simulink model "Dryden"  (R2019b)
settings: Solver=FixedStepAuto  StartTime=0.0  StopTime=1  FixedStep=1  RelTol=1e-3
undefined symbols (not defined in the file): WIND
settings Model: Creator=ibori  LastModifiedBy=Алексей
settings RTWCC: GenCodeOnly=on  PackageGeneratedCodeAndArtifacts=on

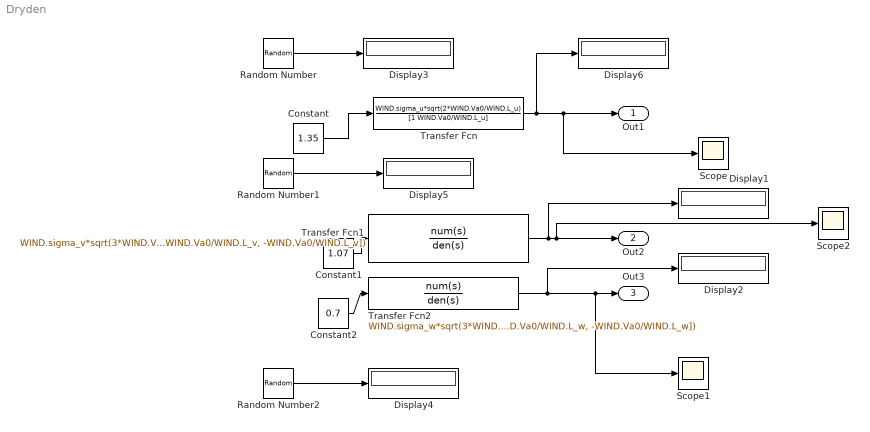
== system Dryden ==
  Constant : Constant  Value=1.35
  Constant1 : Constant  Value=1.07
  Constant2 : Constant  Value=0.7
  Display{1..6} (6 alike) : Display
  Random Number : RandomNumber  SampleTime=1
  Random Number1 : RandomNumber  SampleTime=1
  Random Number2 : RandomNumber  SampleTime=1
  Scope : Scope
  Scope1 : Scope
  Scope2 : Scope
  Transfer Fcn : TransferFcn  Numerator=WIND.sigma_u*sqrt(2*WIND.Va0/WIND.L_u)  Denominator=[1 WIND.Va0/WIND.L_u]
  Transfer Fcn1 : TransferFcn  Numerator=WIND.sigma_v*sqrt(3*WIND.Va0/WIND.L_v)*[0, 1, WIND.Va0/sqrt(3)/WIND.L_v]  Denominator=poly([-WIND.Va0/WIND.L_v, -WIND.Va0/WIND.L_v])
  Transfer Fcn2 : TransferFcn  Numerator=WIND.sigma_w*sqrt(3*WIND.Va0/WIND.L_w)*[0, 1, WIND.Va0/sqrt(3)/WIND.L_w]  Denominator=poly([-WIND.Va0/WIND.L_w, -WIND.Va0/WIND.L_w])
  Out1 : Outport
  Out2 : Outport  Port=2
  Out3 : Outport  Port=3
  wires:
  Random Number/1 -> Display3/1
  Random Number1/1 -> Display5/1
  Random Number2/1 -> Display4/1
  Transfer Fcn/1 -> Display6/1, Scope/1, Out1/1
  Transfer Fcn2/1 -> Display2/1, Scope1/1, Out3/1
  Transfer Fcn1/1 -> Display1/1, Scope2/1, Out2/1
  Constant/1 -> Transfer Fcn/1
  Constant1/1 -> Transfer Fcn1/1
  Constant2/1 -> Transfer Fcn2/1
